simulink model "prosthesis_passivity_adaptive"  (R2017b)
settings: Solver=VariableStepAuto  StartTime=0.0  StopTime=40  FixedStep=0.2  RelTol=1e-3
settings Model: Creator=ArsalanBangash  LastModifiedBy=ArsalanBangash

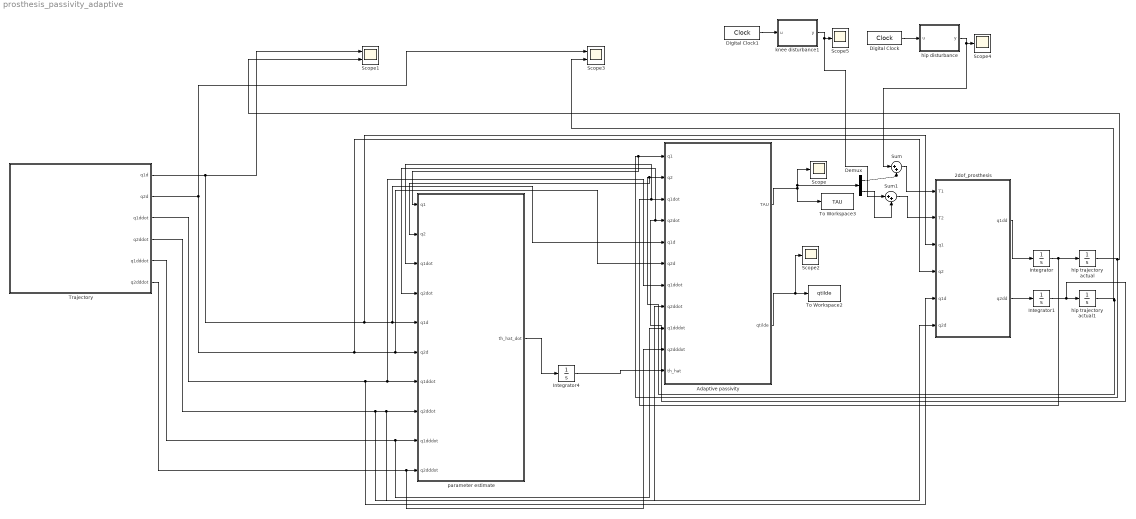
== system prosthesis_passivity_adaptive ==
  2dof_prosthesis : MATLAB Function  TreatAsAtomicUnit=on
  Adaptive passivity : MATLAB Function  TreatAsAtomicUnit=on
  Demux : Demux  Outputs=2
  Digital Clock : DigitalClock
  Digital Clock1 : DigitalClock
  Integrator : Integrator
  Integrator1 : Integrator
  Integrator4 : Integrator
  Scope{,2,4..5} (4 alike) : Scope
  Scope1 : Scope  NumInputPorts=2
  Scope3 : Scope  NumInputPorts=2
  Sum : Sum  Inputs=|++
  Sum1 : Sum  Inputs=|++
  To Workspace2 : ToWorkspace  VariableName=qtilde  SampleTime=-1
  To Workspace3 : ToWorkspace  VariableName=TAU  SampleTime=-1
  Trajectory : Subsystem
  hip disturbance : MATLAB Function  TreatAsAtomicUnit=on
  hip trajectory actual : Integrator
  hip trajectory actual1 : Integrator
  knee disturbance1 : MATLAB Function  TreatAsAtomicUnit=on
  "parameter estimate " : MATLAB Function  TreatAsAtomicUnit=on
  wires:
  Integrator/1 -> "parameter estimate "/3(q1dot), Adaptive passivity/3(q1dot), hip trajectory actual/1
  2dof_prosthesis/1(q1dd) -> Integrator/1
  "parameter estimate "/1(th_hat_dot) -> Integrator4/1
  Integrator4/1 -> Adaptive passivity/11(th_hat)
  Adaptive passivity/1(TAU) -> Demux/1, Scope/1, To Workspace3/1
  Adaptive passivity/2(qtilde) -> Scope2/1, To Workspace2/1
  Trajectory/1(q1d) -> Scope1/1, 2dof_prosthesis/3(q1), Adaptive passivity/5(q1d), "parameter estimate "/5(q1d)
  Trajectory/2(q2d) -> Scope3/1, 2dof_prosthesis/4(q2), Adaptive passivity/6(q2d), "parameter estimate "/6(q2d)
  Trajectory/3(q1ddot) -> 2dof_prosthesis/5(q1d), Adaptive passivity/7(q1ddot), "parameter estimate "/7(q1ddot)
  Trajectory/4(q2ddot) -> 2dof_prosthesis/6(q2d), Adaptive passivity/8(q2ddot), "parameter estimate "/8(q2ddot)
  Trajectory/5(q1dddot) -> Adaptive passivity/9(q1dddot), "parameter estimate "/9(q1dddot)
  Trajectory/6(q2dddot) -> Adaptive passivity/10(q2dddot), "parameter estimate "/10(q2dddot)
  2dof_prosthesis/2(q2dd) -> Integrator1/1
  Integrator1/1 -> "parameter estimate "/4(q2dot), Adaptive passivity/4(q2dot), hip trajectory actual1/1
  hip trajectory actual/1 -> Scope1/2, "parameter estimate "/1(q1), Adaptive passivity/1(q1)
  hip trajectory actual1/1 -> Scope3/2, "parameter estimate "/2(q2), Adaptive passivity/2(q2)
  Demux/1 -> Sum/2
  Sum/1 -> 2dof_prosthesis/1(T1)
  Digital Clock/1 -> hip disturbance/1(u)
  hip disturbance/1(y) -> Scope4/1, Sum/1
  Demux/2 -> Sum1/2
  Sum1/1 -> 2dof_prosthesis/2(T2)
  knee disturbance1/1(y) -> Sum1/1, Scope5/1
  Digital Clock1/1 -> knee disturbance1/1(u)

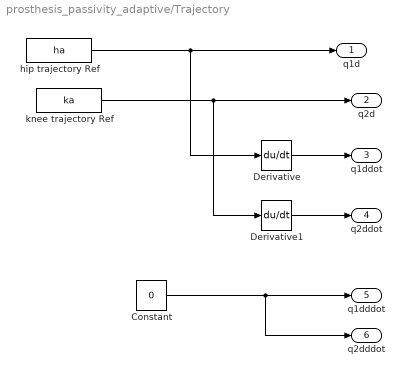
== system prosthesis_passivity_adaptive/Trajectory ==
  Constant : Constant  Value=0
  Derivative : Derivative
  Derivative1 : Derivative
  hip trajectory Ref : FromWorkspace  VariableName=ha  SampleTime=0
  knee trajectory Ref : FromWorkspace  VariableName=ka  SampleTime=0
  q1d : Outport
  q2d : Outport  Port=2
  q1ddot : Outport  Port=3
  q2ddot : Outport  Port=4
  q1dddot : Outport  Port=5
  q2dddot : Outport  Port=6
  wires:
  hip trajectory Ref/1 -> Derivative/1, q1d/1
  knee trajectory Ref/1 -> Derivative1/1, q2d/1
  Derivative/1 -> q1ddot/1
  Derivative1/1 -> q2ddot/1
  Constant/1 -> q2dddot/1, q1dddot/1

== matlab function prosthesis_passivity_adaptive/hip disturbance ==
  data: u input; y output
function y = fcn(u)
time=u;
if (time>10 && time<15)
    y=200;
else
    y=0;
end

== matlab function prosthesis_passivity_adaptive/parameter estimate  ==
  data: q1 input; th_hat_dot output; q2 input; q1dot input; q2dot input; q1d input; q2d input; q1ddot input; q2ddot input; q1dddot input; q2dddot input
function th_hat_dot = parameter_estimator(q1,q2,q1dot,q2dot,q1d,q2d,q1ddot,q2ddot,q1dddot,q2dddot)

Gamma_1=10*eye(5);
g=9.8;

qtilde=[q1-q1d;q2-q2d];
qtildedot=[q1dot-q1ddot;q2dot-q2ddot];

%Gains
L=diag([1 1]);
K=diag([1 1]);

v=[q1ddot;q2ddot]-L*qtilde;
a=[q1dddot;q2dddot]-L*qtildedot;
r=qtildedot+L*qtilde;

%Form the regressor
Y=zeros(2,5);
Y(1,1)=a(1);
Y(1,2)=cos(q2)*(2*a(1)+a(2))-sin(q2)*q2dot*v(1)-sin(q2)*(q1dot+q2dot)*v(2);
Y(1,3)=a(2);
Y(1,4)=g*cos(q1);
Y(1,5)=g*cos(q1+q2);
Y(2,1)=0;
Y(2,2)=cos(q2)*a(1)+sin(q2)*q1dot*v(1);
Y(2,3)=a(1)+a(2);
Y(2,4)=0;
Y(2,5)=Y(1,5);
%y=[Y(1,1) Y(1,2) Y(1,3) Y(1,4) Y(1,5); Y(2,1) Y(2,2) Y(2,3) Y(2,4) Y(2,5)];

th_hat_dot=-Gamma_1*Y'*r;

== matlab function prosthesis_passivity_adaptive/Adaptive passivity ==
  data: q1 input; TAU output; q2 input; q1dot input; q2dot input; q1d input; q2d input; q1ddot input; q2ddot input; q1dddot input; q2dddot input; th_hat input; qtilde output
function [TAU,qtilde]= Adaptive_passivity(q1,q2,q1dot,q2dot,q1d,q2d,q1ddot,q2ddot,q1dddot,q2dddot,th_hat)
%In-class example: 2-link planar RR manipulator

g=9.8;
qtilde=[q1-q1d;q2-q2d];
qtildedot=[q1dot-q1ddot;q2dot-q2ddot];

%Gains
L=diag([1 1]);
K=diag([1 1 ]);

v=[q1ddot;q2ddot]-L*qtilde;
a=[q1dddot;q2dddot]-L*qtildedot;
r=qtildedot+L*qtilde;

%Form the regressor
Y=zeros(2,5);
Y(1,1)=a(1);
Y(1,2)=cos(q2)*(2*a(1)+a(2))-sin(q2)*q2dot*v(1)-sin(q2)*(q1dot+q2dot)*v(2);
Y(1,3)=a(2);
Y(1,4)=g*cos(q1);
Y(1,5)=g*cos(q1+q2);
Y(2,1)=0;
Y(2,2)=cos(q2)*a(1)+sin(q2)*q1dot*v(1);
Y(2,3)=a(1)+a(2);
Y(2,4)=0;
Y(2,5)=Y(1,5);
TAU=(Y*th_hat)-(K*r);

== matlab function prosthesis_passivity_adaptive/2dof_prosthesis ==
  data: T1 input; q1dd output; T2 input; q2dd output; q1 input; q2 input; q1d input; q2d input
function [q1dd,q2dd]= orthosis_hip_knee(T1, T2,q1,q2,q1d,q2d)


m1=1;
m2=1;
l1=1;
l2=1;
g0=9.8;
Ixx1=0.00205024; Ixx2=0.00205024;Iyy1=0.00205024;Iyy2=0.00205024;
Izz1=0.00205024; Izz2=0.00205024;

B=[ Izz1 + Izz2 + 0.25*l1^2*m1 + l1^2*m2 + 0.25*l2^2*m2 + l1*l2*m2*cos(q2), 0.25*m2*l2^2 + 0.5*l1*m2*cos(q2)*l2 + Izz2;
                             0.25*m2*l2^2 + 0.5*l1*m2*cos(q2)*l2 + Izz2,                        0.25*m2*l2^2 + Izz2];


C=[ -0.5*l1*l2*m2*q2d*sin(q2), -(l1*l2*m2*sin(q2)*(q1d + q2d))/2;
  0.5*l1*l2*m2*q1d*sin(q2),                                 0];




 G= [1.0*g0*m2*(0.5*l2*cos(q1 + q2) + 1.0*l1*cos(q1)) + 0.5*g0*l1*m1*cos(q1)
                                               0.5*g0*l2*m2*cos(q1 + q2)];
 


T=[T1;T2];

thd=[q1d;
q2d]

actual_th_dd= inv(B)*(T-C*thd-G);
q1dd= actual_th_dd(1);
q2dd=actual_th_dd(2);

== matlab function prosthesis_passivity_adaptive/knee disturbance1 ==
  data: u input; y output
function y = fcn(u)
time=u;
if (time>20 && time<25)
    y=00;
else
    y=0;
end
